simulink model "estimate_parameters_sim"  (R2019b)
settings: Solver=VariableStepAuto  StartTime=0.0  StopTime=statstop2+1  FixedStep=0.05  RelTol=1e-3
values from neighbouring files (symbols this model uses):
  statstart1 = 30    [estimate_parameters.m]
  statstart2 = 100    [estimate_parameters.m]
  statstop1 = 100    [estimate_parameters.m]
  statstop2 = 170    [estimate_parameters.m]
  stepstop = 10    [estimate_parameters.m]
  umax = 10    [estimate_parameters.m]
  ustat = 7    [estimate_parameters.m]
settings Model: Creator=olle  LastModifiedBy=olle

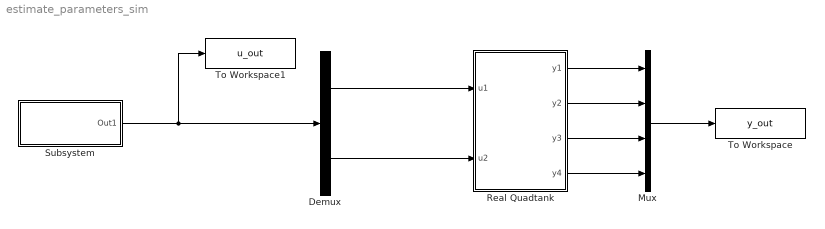
== system estimate_parameters_sim ==
  Demux : Demux  Outputs=2
  Mux : Mux
  Real Quadtank : Subsystem  AncestorBlock=tank/Real Quadtank  VariantControl=Real  mask{h=0.05}
  Subsystem : Subsystem
  To Workspace : ToWorkspace  VariableName=y_out  SaveFormat=Timeseries  SampleTime=-1
  To Workspace1 : ToWorkspace  VariableName=u_out  SaveFormat=Timeseries  SampleTime=-1
  wires:
  Subsystem/1(Out1) -> To Workspace1/1, Demux/1
  Demux/2 -> Real Quadtank/2(u2)
  Demux/1 -> Real Quadtank/1(u1)
  Real Quadtank/3(y3) -> Mux/3
  Real Quadtank/4(y4) -> Mux/4
  Real Quadtank/2(y2) -> Mux/2
  Real Quadtank/1(y1) -> Mux/1
  Mux/1 -> To Workspace/1

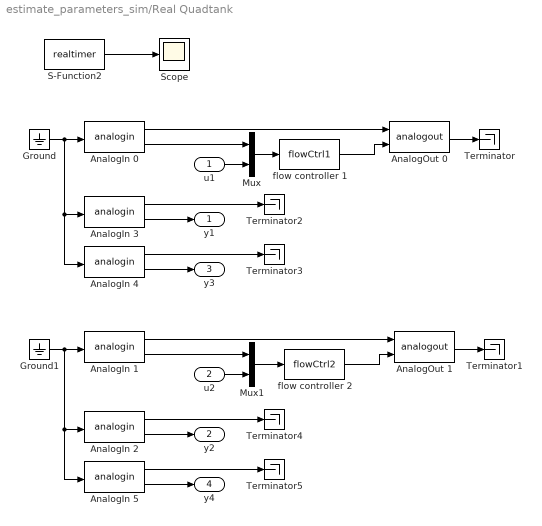
== system estimate_parameters_sim/Real Quadtank ==
  u1 : Inport
  u2 : Inport  Port=2
  AnalogIn 0 : S-Function  FunctionName=analogin  Parameters=h [35]  SFunctionDeploymentMode=off  EnableBusSupport=off
  AnalogIn 1 : S-Function  FunctionName=analogin  Parameters=h [34]  SFunctionDeploymentMode=off  EnableBusSupport=off
  AnalogIn 2 : S-Function  FunctionName=analogin  Parameters=h [33]  SFunctionDeploymentMode=off  EnableBusSupport=off
  AnalogIn 3 : S-Function  FunctionName=analogin  Parameters=h [31]  SFunctionDeploymentMode=off  EnableBusSupport=off
  AnalogIn 4 : S-Function  FunctionName=analogin  Parameters=h [30]  SFunctionDeploymentMode=off  EnableBusSupport=off
  AnalogIn 5 : S-Function  FunctionName=analogin  Parameters=h [32]  SFunctionDeploymentMode=off  EnableBusSupport=off
  AnalogOut 0 : S-Function  FunctionName=analogout  Parameters=h [31]  SFunctionDeploymentMode=off  EnableBusSupport=off
  AnalogOut 1 : S-Function  FunctionName=analogout  Parameters=h [30]  SFunctionDeploymentMode=off  EnableBusSupport=off
  Ground : Ground
  Ground1 : Ground
  Mux : Mux  Inputs=2
  Mux1 : Mux  Inputs=2
  S-Function2 : S-Function  FunctionName=realtimer  Parameters=h  SFunctionDeploymentMode=off  EnableBusSupport=off
  Scope : Scope
  Terminator{,1..5} (6 alike) : Terminator
  flow controller 1 : MATLABFcn  MATLABFcn=flowCtrl1  SampleTime=0.01
  flow controller 2 : MATLABFcn  MATLABFcn=flowCtrl2  SampleTime=0.01
  y1 : Outport
  y2 : Outport  Port=2
  y3 : Outport  Port=3
  y4 : Outport  Port=4
  wires:
  AnalogIn 0/2 -> Mux/1
  AnalogIn 1/2 -> Mux1/1
  flow controller 2/1 -> AnalogOut 1/2
  Mux1/1 -> flow controller 2/1
  u2/1 -> Mux1/2
  flow controller 1/1 -> AnalogOut 0/2
  Mux/1 -> flow controller 1/1
  u1/1 -> Mux/2
  AnalogIn 5/1 -> Terminator5/1
  AnalogIn 2/1 -> Terminator4/1
  Ground1/1 -> AnalogIn 1/1, AnalogIn 2/1, AnalogIn 5/1
  AnalogIn 5/2 -> y4/1
  AnalogIn 2/2 -> y2/1
  AnalogIn 4/1 -> Terminator3/1
  AnalogIn 3/1 -> Terminator2/1
  Ground/1 -> AnalogIn 4/1, AnalogIn 3/1, AnalogIn 0/1
  AnalogIn 4/2 -> y3/1
  AnalogIn 3/2 -> y1/1
  AnalogOut 1/1 -> Terminator1/1
  AnalogIn 1/1 -> AnalogOut 1/1
  AnalogOut 0/1 -> Terminator/1
  AnalogIn 0/1 -> AnalogOut 0/1
  S-Function2/1 -> Scope/1

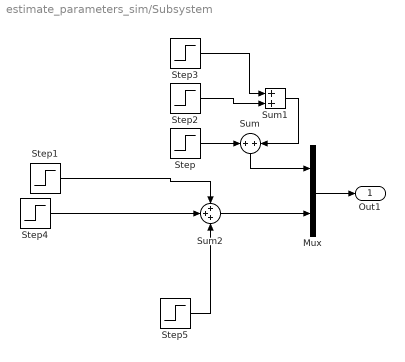
== system estimate_parameters_sim/Subsystem ==
  Mux : Mux  Inputs=2
  Step : Step  Time=stepstop  Before=umax  After=0  SampleTime=0.05
  Step1 : Step  Time=statstart2  After=ustat  SampleTime=0
  Step2 : Step  Time=statstart1  After=ustat  SampleTime=0.05
  Step3 : Step  Time=statstop1  After=-ustat  SampleTime=0.05
  Step4 : Step  Time=statstop2  After=-ustat  SampleTime=0
  Step5 : Step  Time=stepstop  Before=umax  After=0  SampleTime=0.05
  Sum : Sum  Inputs=2
  Sum1 : Sum
  Sum2 : Sum  Inputs=3
  Out1 : Outport
  wires:
  Sum/1 -> Mux/1
  Step/1 -> Sum/1
  Mux/1 -> Out1/1
  Sum1/1 -> Sum/2
  Step2/1 -> Sum1/2
  Step3/1 -> Sum1/1
  Step1/1 -> Sum2/1
  Step4/1 -> Sum2/2
  Sum2/1 -> Mux/2
  Step5/1 -> Sum2/3
